simulink model "clase_008_codigo_002"  (R2024a)
settings: Solver=VariableStepAuto  StartTime=0.0  StopTime=1  RelTol=1e-3

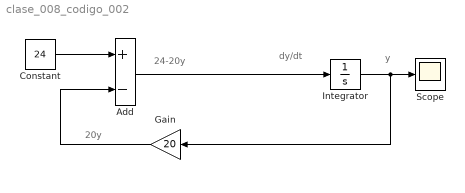
== system clase_008_codigo_002 ==
  note: 24-20y
  note: 20y
  note: dy/dt
  note: y
  Add : Sum  Inputs=+-
  Constant : Constant  Value=24
  Gain : Gain  Gain=20
  Integrator : Integrator
  Scope : Scope
  wires:
  Integrator/1 -> Gain/1, Scope/1
  Constant/1 -> Add/1
  Gain/1 -> Add/2
  Add/1 -> Integrator/1
